simulink model "orbit_simulation"  (R2025a)
settings: Solver=ode4  StartTime=0.0  StopTime=t_stop  FixedStep=1  RelTol=1e-3
values from neighbouring files (symbols this model uses):
  dec_year = 2025.0    (= 2025)    [orbit_test.m]
  degree = 13    [orbit_test.m]
undefined symbols (not defined in the file or in its folder): C_nm, IAU, juliandate
libraries: aerolibtransform2 x1
settings Model: Creator=Guilherme  LastModifiedBy=Guilherme

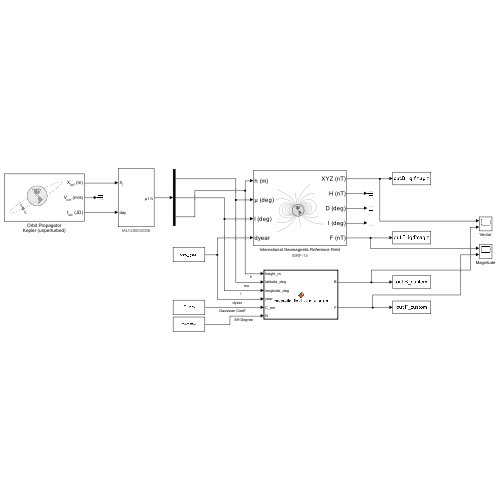
[thumbnail: Simulink's stored preview of the top-level diagram]
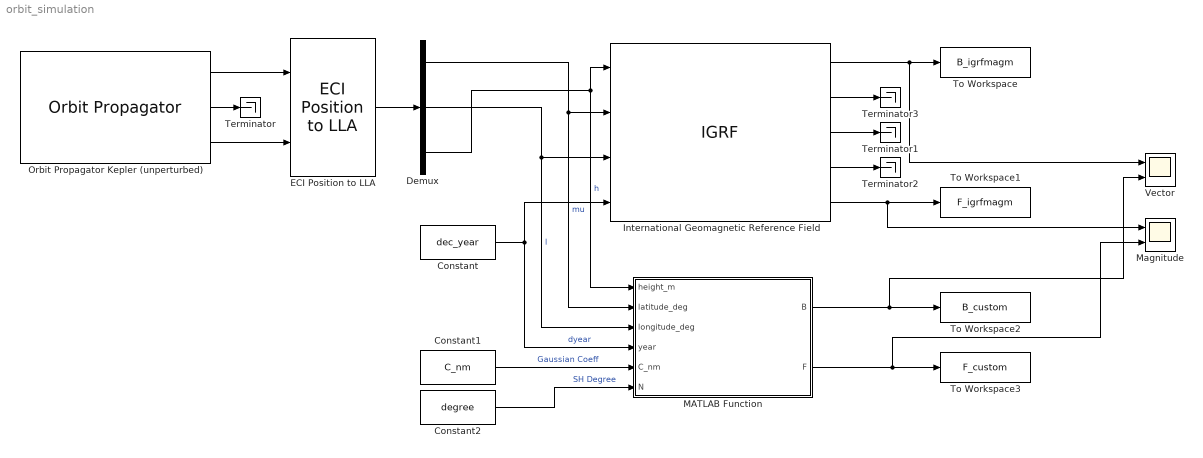
== system orbit_simulation ==
  Constant : Constant  Value=dec_year
  Constant1 : Constant  Value=C_nm
  Constant2 : Constant  Value=degree
  Demux : Demux  Outputs=3
  ECI Position to LLA : aerolibtransform2/ECI Position to LLA  red=IAU-2000/2006  year=2025  month=January  day=1  hour=0  min=0  sec=0  deltaT=Day  errorflag=Error  extraparamflag=off  eunits=Metric (MKS)  earthmodel=WGS84  flat=1/298.257223563  eqradius=6378137
      settings: AttributesFormatString=%<red>
  International Geomagnetic Reference Field : IGRF  month=January  day=1  sv_out=off
      settings: AttributesFormatString=%<generation>
  MATLAB Function : MATLAB Function  TreatAsAtomicUnit=on
  Magnitude : Scope  NumInputPorts=2
      settings: ActiveDisplayYMinimum=11577.907288855116  ActiveDisplayYMaximum=45556.752301250141
  Orbit Propagator Kepler (unperturbed) : OrbitPropagator  startDate=juliandate(2025, 1, 1, 12, 0, 0)  semiMajorAxis=a  eccentricity=e  inclination=inc  raan=RAAN  argPeriapsis=omega  trueAnomaly=nu  inertialPosition=[3649700.0 3308200.0 -4676600.0]  inertialVelocity=[-2750.8 6666.4 2573.4]  fixedPosition=[-4142689.0 -2676864.7 -4669861.6]  fixedVelocity=[1452.7 -6720.7 2568.1]  customR=3396200  customMu=4.305e13  customJ2=1.0826269e-03  customOmega=4.06125949e-3
  Terminator{,1..3} (4 alike) : Terminator
  To Workspace : ToWorkspace  VariableName=B_igrfmagm  SaveFormat=Timeseries  SampleTime=-1
  To Workspace1 : ToWorkspace  VariableName=F_igrfmagm  SaveFormat=Timeseries  SampleTime=-1
  To Workspace2 : ToWorkspace  VariableName=B_custom  SaveFormat=Timeseries  SampleTime=-1
  To Workspace3 : ToWorkspace  VariableName=F_custom  SaveFormat=Timeseries  SampleTime=-1
  Vector : Scope  NumInputPorts=2
      settings: ActiveDisplayYMinimum=-29314.633715673495  ActiveDisplayYMaximum=40392.322261246925
  wires:
  Orbit Propagator Kepler (unperturbed)/1 -> ECI Position to LLA/1
  Orbit Propagator Kepler (unperturbed)/2 -> Terminator/1
  ECI Position to LLA/1 -> Demux/1
  Orbit Propagator Kepler (unperturbed)/3 -> ECI Position to LLA/2
  Demux/3 -> International Geomagnetic Reference Field/1, MATLAB Function/1(height_m)  "h"
  Demux/1 -> International Geomagnetic Reference Field/2, MATLAB Function/2(latitude_deg)  "mu"
  Demux/2 -> International Geomagnetic Reference Field/3, MATLAB Function/3(longitude_deg)  "l"
  Constant/1 -> International Geomagnetic Reference Field/4, MATLAB Function/4(year)  "dyear"
  International Geomagnetic Reference Field/3 -> Terminator1/1
  International Geomagnetic Reference Field/4 -> Terminator2/1
  International Geomagnetic Reference Field/2 -> Terminator3/1
  International Geomagnetic Reference Field/1 -> Vector/1, To Workspace/1
  International Geomagnetic Reference Field/5 -> Magnitude/1, To Workspace1/1
  Constant1/1 -> MATLAB Function/5(C_nm)  "Gaussian Coeff"
  Constant2/1 -> MATLAB Function/6(N)  "SH Degree"
  MATLAB Function/1(B) -> Vector/2, To Workspace2/1
  MATLAB Function/2(F) -> Magnitude/2, To Workspace3/1

== matlab function orbit_simulation/MATLAB Function ==
  data: height_m input; B output; latitude_deg input; longitude_deg input; year input; C_nm input; N input; F output
function [B, F] = magnetic_field_computation(height_m, latitude_deg, longitude_deg, year, C_nm, N)

    [B, F] = magnetic_field(height_m, latitude_deg, longitude_deg, year, C_nm, N);

end
